simulink model "SpringMassDamper_PID"  (R2021a)
settings: Solver=FixedStepAuto  StartTime=0.0  StopTime=50.0  FixedStep=0.1  RelTol=1e-3
values from neighbouring files (symbols this model uses):
  b = Simulink.Parameter    [init.m]
  k = Simulink.Parameter    [init.m]
  Kd = Simulink.Parameter    [init.m]
  Ki = Simulink.Parameter    [init.m]
  Kp = Simulink.Parameter    [init.m]
  m = Simulink.Parameter    [init.m]
settings Model: Creator=matthias  LastModifiedBy=matthias
settings DataIOCC: SaveOutput=off  SignalLogging=off  DSMLogging=off  SaveTime=off  ReturnWorkspaceOutputs=off
settings HardwareCC: TargetBitPerLong=64  TargetBitPerPointer=64  TargetBitPerSizeT=64  TargetBitPerPtrDiffT=64  TargetLongLongMode=on  TargetIntDivRoundTo=Zero  TargetEndianess=LittleEndian  TargetWordSize=64  TargetHWDeviceType=MATLAB Host  ProdEqTarget=off
settings RTWCC: Description=Generic Real-Time Target  GenCodeOnly=on  PackageGeneratedCodeAndArtifacts=on  PackageName=pidsmd-union  RTWVerbose=off
settings GRTTargetCC: MatFileLogging=off

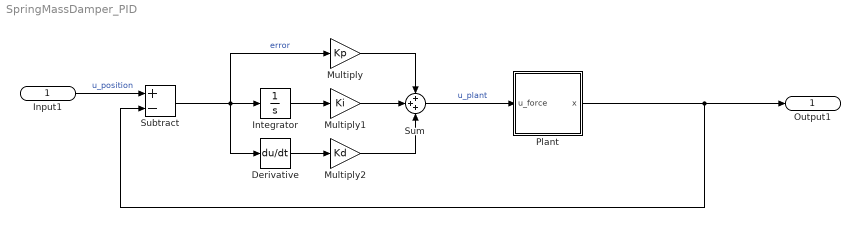
== system SpringMassDamper_PID ==
  Input1 : Inport
  Derivative : Derivative
  Integrator : Integrator
  Multiply : Gain  Gain=Kp
  Multiply1 : Gain  Gain=Ki
  Multiply2 : Gain  Gain=Kd
  Plant : Subsystem
  Subtract : Sum  Inputs=+-
  Sum : Sum  Inputs=+++
  Output1 : Outport  SignalName=position
  wires:
  Plant/1(x) -> Output1/1, Subtract/2
  Subtract/1 -> Derivative/1, Integrator/1, Multiply/1  "error"
  Integrator/1 -> Multiply1/1
  Multiply1/1 -> Sum/2
  Multiply/1 -> Sum/1
  Sum/1 -> Plant/1(u_force)  "u_plant"
  Input1/1 -> Subtract/1  "u_position"
  Derivative/1 -> Multiply2/1
  Multiply2/1 -> Sum/3

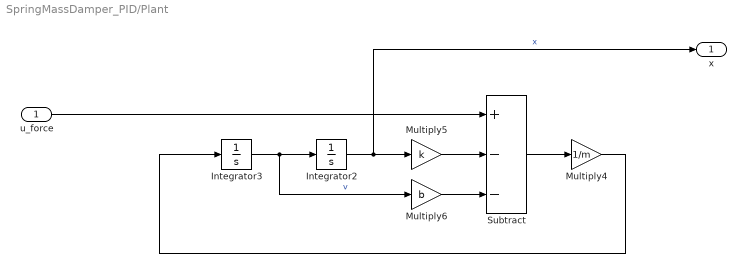
== system SpringMassDamper_PID/Plant ==
  u_force : Inport
  Integrator2 : Integrator
  Integrator3 : Integrator
  Multiply4 : Gain  Gain=1/m
  Multiply5 : Gain  Gain=k
  Multiply6 : Gain  Gain=b
  Subtract : Sum  Inputs=+--
  x : Outport
  wires:
  u_force/1 -> Subtract/1
  Subtract/1 -> Multiply4/1
  Multiply5/1 -> Subtract/2
  Multiply6/1 -> Subtract/3
  Multiply4/1 -> Integrator3/1
  Integrator3/1 -> Multiply6/1, Integrator2/1  "v"
  Integrator2/1 -> x/1, Multiply5/1  "x"
